simulink model "signals1"  (R2019b)
settings: Solver=VariableStepAuto  StartTime=0.0  StopTime=10.0  RelTol=1e-3
model workspace (MAT data in the model file):
  Amp = 1
libraries: simulink x5
settings Model: OrderedModelArguments=off  Creator=HUAWEI  LastModifiedBy=HUAWEI

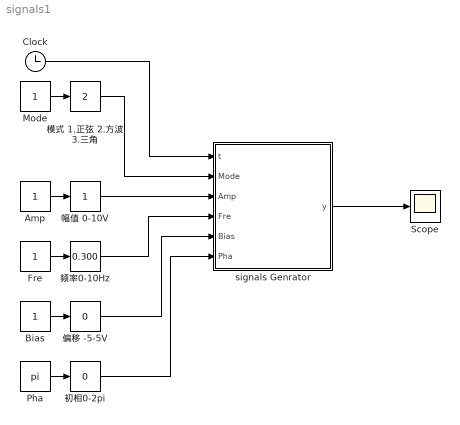
== system signals1 ==
  Amp : Constant  OutMin=[0]  OutMax=[10]
  Bias : Constant  OutMin=[-5]  OutMax=[5]
  Clock : Clock
  Fre : Constant  OutMin=[0]  OutMax=[10]
  Mode : Constant
  Pha : Constant  Value=pi  OutMin=[0]  OutMax=[2*pi]
  Scope : Scope
  signals Genrator : MATLAB Function  TreatAsAtomicUnit=on
  偏移 -5-5V : simulink/Math Operations/Slider Gain  gain=0  low=-5  high=5
  初相0-2pi : simulink/Math Operations/Slider Gain  gain=0  low=0  high=2
  幅值 0-10V : simulink/Math Operations/Slider Gain  gain=1  low=0  high=10
  模式 1.正弦 2.方波 3.三角 : simulink/Math Operations/Slider Gain  gain=2  low=1  high=3
  频率0-10Hz : simulink/Math Operations/Slider Gain  gain=0.300  low=0  high=10
  wires:
  Clock/1 -> signals Genrator/1(t)
  Mode/1 -> 模式 1.正弦 2.方波 3.三角/1
  Pha/1 -> 初相0-2pi/1
  Bias/1 -> 偏移 -5-5V/1
  Fre/1 -> 频率0-10Hz/1
  幅值 0-10V/1 -> signals Genrator/3(Amp)
  signals Genrator/1(y) -> Scope/1
  模式 1.正弦 2.方波 3.三角/1 -> signals Genrator/2(Mode)
  频率0-10Hz/1 -> signals Genrator/4(Fre)
  偏移 -5-5V/1 -> signals Genrator/5(Bias)
  初相0-2pi/1 -> signals Genrator/6(Pha)
  Amp/1 -> 幅值 0-10V/1

== matlab function signals1/signals Genrator ==
  data: t input; y output; Mode input; Amp input; Fre input; Bias input; Pha input
% @discription: different types of signal generator function
% @Author：Zhang Yifan
% @date:2020-4-17 16:28
function y = fcn(t,Mode,Amp,Fre,Bias,Pha)
%产生周期性待调制的锯齿波 范围-pi至pi
temp = mod(2*pi*Fre*t+Pha,2*pi)-pi;
if Mode == 1
    y = Amp*sin(temp)+Bias;
elseif Mode == 2
    y = Amp*sign(sin(temp))+Bias;
elseif Mode == 3
    y = Amp*(abs(temp)-pi/2)/(pi/2)+Bias;
else
    y = 0;
end
